simulink model "All_Controllers_Sim"  (R2023b)
settings: Solver=FixedStepDiscrete  StartTime=0.0  StopTime=0.5  FixedStep=0.001  RelTol=1e-3  EnableMultiTasking=on
PostLoadFcn:
  | , if any(exist('dsrtsu_mdlpostloadfcn', 'file') == [2, 3, 6]), try dsrtsu_mdlpostloadfcn('Execute', bdroot); catch fprintf('Error in PostLoadFcn (dsrtsu_mdlpostloadfcn) for model "%s":\n %s\n', bdroot, lasterr); end, end,
values from neighbouring files (symbols this model uses):
  A = [r, A(len_B+1:end)]    [All_Controllers.m]
  B = [0.7585 -0.4552]    [All_Controllers.m]
  C = [x, C_next]    [All_Controllers.m]
  D = [0, D_next]    [All_Controllers.m]
  plant_delay = 5    [All_Controllers.m]
  R = conv(H, F)    [All_Controllers.m]
  S = S1 + S2    [All_Controllers.m]
  T = conv(H, C)    [All_Controllers.m]
libraries: simulink x2
settings Model: DSRTSU_INTERNAL_RTI_VER=460  DSRTSU_INTERNAL_RTI_TYPE=rti1401  DSRTSU_INTERNAL_RTIFPGA=50  Creator=jreuter  LastModifiedBy=jonasbechler
settings SolverCC: AlgebraicLoopSolver=TrustRegion
settings DataIOCC: SaveFormat=Array  ReturnWorkspaceOutputs=off
settings OptimizationCC: BlockReduction=off  OptimizeBlockIOStorage=off  BufferReuse=off  GlobalBufferReuse=off  ExpressionFolding=off  LocalBlockOutputs=off  LifeSpan=inf
settings DebuggingCC: UnconnectedInputMsg=warning  UnconnectedOutputMsg=warning  UnconnectedLineMsg=warning  SFUnexpectedBacktrackingDiag=warning  SFNoUnconditionalDefaultTransitionDiag=warning  SFExecutionAtInitializationDiag=none  ArithmeticOperatorsInVariantConditions=warning
settings HardwareCC: ProdBitPerPointer=32  ProdBitPerSizeT=32  ProdBitPerPtrDiffT=32  ProdLargestAtomicFloat=None  ProdEndianess=BigEndian  ProdWordSize=32  ProdHWDeviceType=Generic->Custom  TargetIntDivRoundTo=Zero  TargetEndianess=BigEndian  TargetHWDeviceType=Generic->Custom
settings ModelReferenceCC: EnableRefExpFcnMdlSchedulingChecks=on  PropagateSignalLabelsOutOfModel=off
settings SFSimCC: SimUseLocalCustomCode=off  CustomCodeUndefinedFunction=UseInterfaceOnly
settings RTWCC: Description=dSPACE DS1104 Hardware Platform  SystemTargetFile=rti1104.tlc  MakeCommand=make_rti  TemplateMakefile=rti1104.tmf  RTWUseLocalCustomCode=off  DLArmComputeVersion=19.05
settings CodeAppCC: StateflowObjectComments=on
settings STFCustomTargetCC: TargetLangStandard=C89/C90 (ANSI)  ParMdlRefBuildCompliant=on  MatFileLogging=on  GRTInterface=on  SystemTargetFile=rti1104.tlc
settings GRTTargetCC: TargetLangStandard=C89/C90 (ANSI)  CompOptLevelCompliant=off  ConcurrentExecutionCompliant=off  CombineOutputUpdateFcns=off  CPPClassGenCompliant=off  GRTInterface=on  UseToolchainInfoCompliant=off  ExtModeMexFile=noextcomm
settings ConfigComp: CovMetricSettings=dw  CovSaveCumulativeToWorkspaceVar=on  CovSaveSingleToWorkspaceVar=on  CovExternalEMLEnable=off

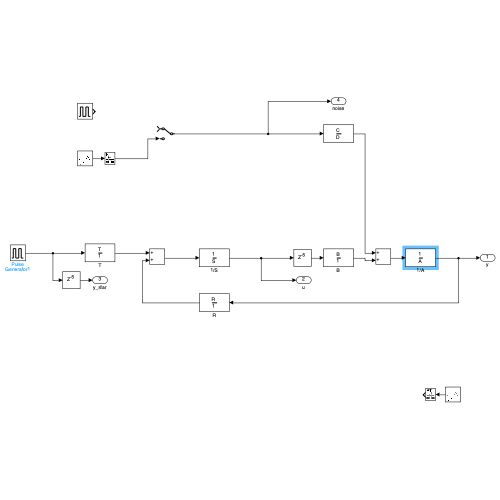
[thumbnail: Simulink's stored preview of the top-level diagram]
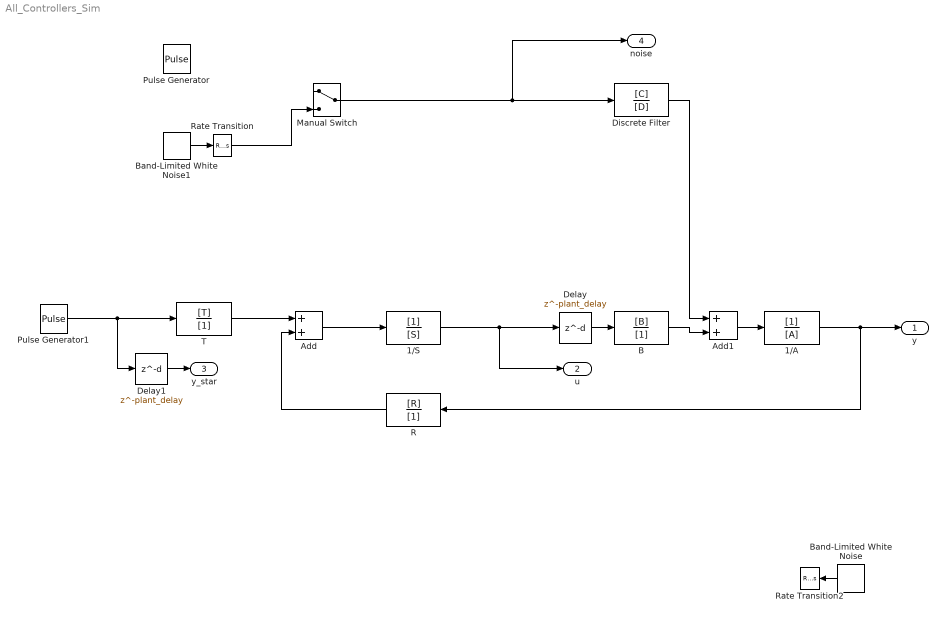
== system All_Controllers_Sim ==
  1/A : DiscreteFilter  Denominator=[A]
  1/S : DiscreteFilter  Denominator=[S]
  Add : Sum
  Add1 : Sum
  B : DiscreteFilter  Numerator=[B]  Denominator=[1]
  Band-Limited White Noise : simulink/Sources/Band-Limited White Noise  Cov=1e-9  Ts=.1  seed=[23341]
  Band-Limited White Noise1 : simulink/Sources/Band-Limited White Noise  Cov=0.1  Ts=.1  seed=[23341]
  Delay : Delay  DelayLength=plant_delay  InitialCondition=0
  Delay1 : Delay  DelayLength=plant_delay  InitialCondition=0
  Discrete Filter : DiscreteFilter  Numerator=[C]  Denominator=[D]
  Manual Switch : ManualSwitch
  Pulse Generator : DiscretePulseGenerator  PulseType=Time based  Amplitude=0.1  Period=1  PulseWidth=50
  Pulse Generator1 : DiscretePulseGenerator  PulseType=Time based  Amplitude=10  Period=0.1  PulseWidth=50
  R : DiscreteFilter  Numerator=[R]  Denominator=[1]
  Rate Transition : RateTransition  Integrity=off  OutPortSampleTimeOpt=Inherit
  Rate Transition2 : RateTransition  Integrity=off  OutPortSampleTimeOpt=Inherit
  T : DiscreteFilter  Numerator=[T]  Denominator=[1]
  y : Outport
  u : Outport  Port=2
  y_star : Outport  Port=3
  noise : Outport  Port=4
  wires:
  Band-Limited White Noise1/1 -> Rate Transition/1
  Band-Limited White Noise/1 -> Rate Transition2/1
  Delay/1 -> B/1
  Manual Switch/1 -> Discrete Filter/1, noise/1
  Add/1 -> 1/S/1
  Pulse Generator1/1 -> Delay1/1, T/1
  R/1 -> Add/2
  1/S/1 -> u/1, Delay/1
  B/1 -> Add1/2
  Rate Transition/1 -> Manual Switch/2
  1/A/1 -> R/1, y/1
  T/1 -> Add/1
  Add1/1 -> 1/A/1
  Discrete Filter/1 -> Add1/1
  Delay1/1 -> y_star/1
